simulink model "adaptive_control"  (R2019a)
settings: Solver=VariableStepAuto  StartTime=0.0  StopTime=50  RelTol=1e-3
values from neighbouring files (symbols this model uses):
  alphap = -3*[0.01 -1 1 0.5]'    [main.m]
  am = -4    [main.m]
  f_plant = @(x,u) ap * x + kp * u + alphap' * fz(x)    [main.m]
  fz = @(x) [x^3 exp(-10*(x+0.5)^2) exp(-10*(x-0.5)^2) sin(2*x)]'    [main.m]
  gamma = 2    [main.m]
  km = 4    [main.m]
  kp = 3    [main.m]
  theta_0 = zeros( size(ap,1) + size(kp,2) + size(alphap,1),1)    [main.m]
  theta_true = [km/kp; (am-ap)/kp; -alphap/kp]    [main.m]
  xm_0 = 0    [main.m]
  xp_0 = 0    [main.m]
libraries: dspsrcs4 x1
settings Model: OrderedModelArguments=off  Creator=lucas  LastModifiedBy=lucas

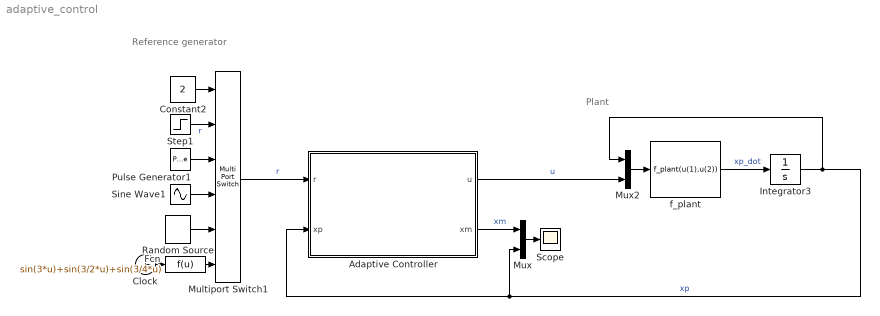
== system adaptive_control ==
  note: Reference generator
  note: Plant
  Adaptive Controller : Subsystem
  Clock : Clock
  Constant2 : Constant  Value=2
  Fcn : Fcn  Expr=sin(3*u)+sin(3/2*u)+sin(3/4*u)
  Integrator3 : Integrator  InitialCondition=xp_0
  Multiport Switch1 : MultiPortSwitch  Inputs=5
  Mux : Mux  Inputs=2
  Mux2 : Mux  Inputs=2
  Pulse Generator1 : DiscretePulseGenerator  PulseType=Time based  Amplitude=4  Period=3  PulseWidth=50
  Random Source : dspsrcs4/Random Source  SrcType=Uniform  NormMethod=Ziggurat  CltLength=12  MinVal=-4  MaxVal=4  MeanVal=0  VarVal=1  RepMode=Not repeatable  rawSeed=1  IsInherit=off  SampMode=Discrete  SampTime=1  SampFrame=1  DataType=Double  OutComplex=Real  OutputFrames=off
  Scope : Scope
  Sine Wave1 : Sin  Amplitude=4  Frequency=0.1  SampleTime=0
  Step1 : Step  After=4  SampleTime=0
  f_plant : MATLABFcn  MATLABFcn=f_plant(u(1),u(2))  OutputDimensions=1
  wires:
  Sine Wave1/1 -> Multiport Switch1/4
  Constant2/1 -> Multiport Switch1/1
  Pulse Generator1/1 -> Multiport Switch1/3
  Multiport Switch1/1 -> Adaptive Controller/1(r)  "r"
  Step1/1 -> Multiport Switch1/2  "r"
  Integrator3/1 -> Mux2/1, Mux/2, Adaptive Controller/2(xp)  "xp"
  Adaptive Controller/1(u) -> Mux2/2  "u"
  f_plant/1 -> Integrator3/1  "xp_dot"
  Mux2/1 -> f_plant/1
  Adaptive Controller/2(xm) -> Mux/1  "xm"
  Mux/1 -> Scope/1
  Random Source/1 -> Multiport Switch1/5
  Fcn/1 -> Multiport Switch1/6
  Clock/1 -> Fcn/1

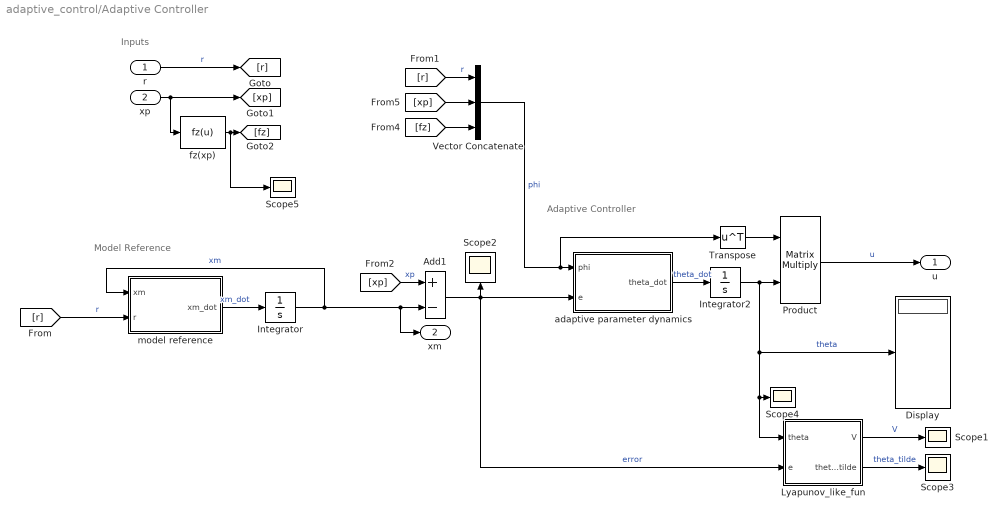
== system adaptive_control/Adaptive Controller ==
  note: Inputs
  note: Model Reference
  note: Adaptive Controller
  r : Inport
  xp : Inport  Port=2
  Add1 : Sum  Inputs=+-
  Display : Display
  Integrator : Integrator  InitialCondition=xm_0
  Integrator2 : Integrator  InitialCondition=theta_0
  Lyapunov_like_fun : MATLAB Function  TreatAsAtomicUnit=on
  Product : Product  Multiplication=Matrix(*)
  Scope{1..5} (5 alike) : Scope
  Transpose : Math  Operator=transpose  SaturateOnIntegerOverflow=on
  Vector Concatenate : Concatenate  NumInputs=3
  adaptive parameter dynamics : MATLAB Function  TreatAsAtomicUnit=on
  fz(xp) : MATLABFcn  MATLABFcn=fz(u)  OutputDimensions=length(alphap)
  model reference : MATLAB Function  TreatAsAtomicUnit=on
  u : Outport
  xm : Outport  Port=2
  wires:
  Vector Concatenate/1 -> Transpose/1, adaptive parameter dynamics/1(phi)  "phi"
  adaptive parameter dynamics/1(theta_dot) -> Integrator2/1  "theta_dot"
  Transpose/1 -> Product/1
  model reference/1(xm_dot) -> Integrator/1  "xm_dot"
  Integrator/1 -> xm/1, Add1/2, model reference/1(xm)  "xm"
  [fz] -> Vector Concatenate/3
  Add1/1 -> adaptive parameter dynamics/2(e), Lyapunov_like_fun/2(e), Scope2/1  "error"
  Lyapunov_like_fun/1(V) -> Scope1/1  "V"
  Lyapunov_like_fun/2(theta_tilde) -> Scope3/1  "theta_tilde"
  Integrator2/1 -> Display/1, Scope4/1, Lyapunov_like_fun/1(theta), Product/2  "theta"
  Product/1 -> u/1  "u"
  [r] -> model reference/2(r)  "r"
  r/1 -> [r]  "r"
  [r] -> Vector Concatenate/1  "r"
  xp/1 -> fz(xp)/1, [xp]
  [xp] -> Add1/1  "xp"
  fz(xp)/1 -> Scope5/1, [fz]
  [xp] -> Vector Concatenate/2

== matlab function adaptive_control/Adaptive Controller/Lyapunov_like_fun ==
  data: theta input; e input; V output; kp parameter; gamma parameter; theta_true parameter; theta_tilde output
function [V,theta_tilde] = Lyap_fun(theta, e, kp, gamma, theta_true)
    
    V = zeros(1);
    theta_tilde = theta_true - theta;
    V = 1/2 * e^2 + 1/2 * abs(kp) *(theta_tilde' / gamma * theta_tilde);

== matlab function adaptive_control/Adaptive Controller/adaptive parameter dynamics ==
  data: phi input; theta_dot output; e input size=1; kp parameter; gamma parameter
function theta_dot = fcn(phi, e, kp, gamma)

    theta_dot = - gamma * sign(kp) * phi * e;
    
%     theta_dot([3,6]) = 0;

== matlab function adaptive_control/Adaptive Controller/model reference ==
  data: xm input; r input; xm_dot output; am parameter; km parameter
function xm_dot = fcn(xm, r, am, km)

    xm_dot = am * xm + km * r;
